simulink model "AAI"  (R2022a)
settings: Solver=FixedStepAuto  StartTime=0.0  StopTime=10.0  FixedStep=1e-3  RelTol=1e-3  EnableMultiTasking=on
undefined symbols (not defined in the file): D0, D10, D11, D12, D13, D2, D4, D5, D6, D7, D8, D9, PTA0, PTA2, PTB23, PTB9, PTC16, PTC2, PTC3, PTC4, PTD0, PTD1, PTD2, PTD3
libraries: frdmk64flib x12
settings Model: ExtModeTrigDuration=5  Creator=ethan  LastModifiedBy=taimu
settings OptimizationCC: EnhancedBackFolding=on  PassReuseOutputArgsAs=Individual arguments  ZeroExternalMemoryAtStartup=off  ZeroInternalMemoryAtStartup=off  MaxStackSize=64  OptimizeBlockOrder=speed  DifferentSizesBufferReuse=on  OptimizationCustomize=off  EfficientTunableParamExpr=on
settings DebuggingCC: ParameterTunabilityLossMsg=error
settings HardwareCC: ProdBitPerPointer=32  ProdBitPerSizeT=32  ProdBitPerPtrDiffT=32  ProdLargestAtomicInteger=Long  ProdLargestAtomicFloat=Double  ProdWordSize=32  ProdHWDeviceType=ARM Compatible->ARM Cortex
settings SFSimCC: MATLABDynamicMemAlloc=off
settings RTWCC: SystemTargetFile=ert.tlc  HardwareBoard=NXP FRDM-K64F  TLCOptions="-aInlineSetEventsForThisBaseRateFcn=TLC_FALSE -aSuppressMultiTaskScheduler=TLC_FALSE  -aRateBasedStepFcn=0"  TemplateMakefile=ert_default_tmf  Toolchain=GNU Tools for ARM Embedded Processors
settings CodeAppCC: ForceParamTrailComments=on  IgnoreCustomStorageClasses=off  OperatorAnnotations=on  SimulinkDataObjDesc=on  SFDataObjDesc=on  InsertBlockDesc=on
settings ERTTargetCC: ExtModeTransport=4  ExtModeMexFile=sendToCommService

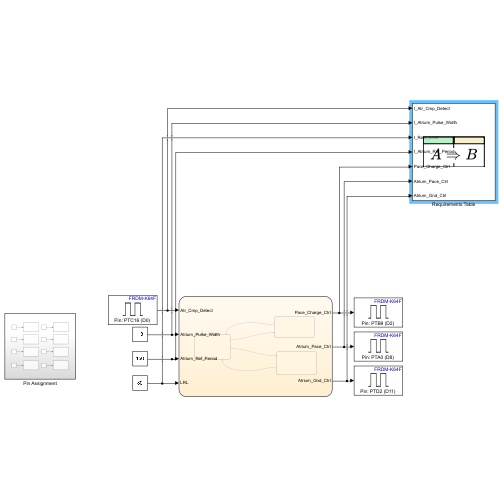
[thumbnail: Simulink's stored preview of the top-level diagram]
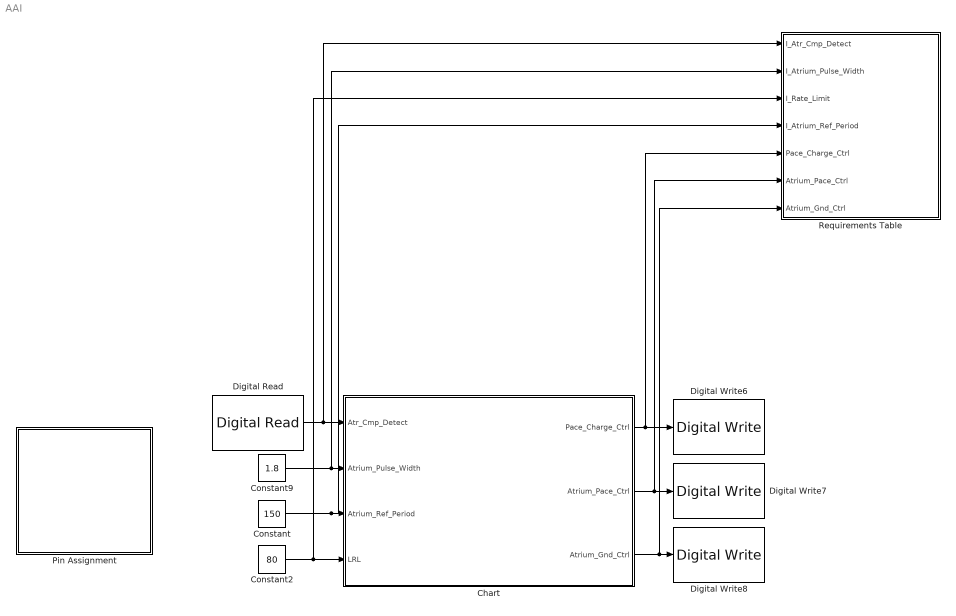
== system AAI ==
  Chart : Stateflow chart  TreatAsAtomicUnit=on
  Constant : Constant  Value=150  OutDataTypeStr=int16
  Constant2 : Constant  Value=80
  Constant9 : Constant  Value=1.8
  Digital Read : frdmk64flib/Digital Read  Whichpin=PTC16 (D0)  SampleTime=-1
  Digital Write6 : frdmk64flib/Digital Write  Whichpin=PTB9 (D2)
  Digital Write7 : frdmk64flib/Digital Write  Whichpin=PTA0 (D8)
  Digital Write8 : frdmk64flib/Digital Write  Whichpin=PTD2 (D11)
  Pin Assignment : Subsystem
  Requirements Table : Requirements Table  TreatAsAtomicUnit=on
  wires:
  Chart/3(Atrium_Gnd_Ctrl) -> Requirements Table/7(Atrium_Gnd_Ctrl), Digital Write8/1
  Chart/2(Atrium_Pace_Ctrl) -> Requirements Table/6(Atrium_Pace_Ctrl), Digital Write7/1
  Constant2/1 -> Requirements Table/3(I_Rate_Limit), Chart/4(LRL)
  Constant9/1 -> Requirements Table/2(I_Atrium_Pulse_Width), Chart/2(Atrium_Pulse_Width)
  Chart/1(Pace_Charge_Ctrl) -> Requirements Table/5(Pace_Charge_Ctrl), Digital Write6/1
  Digital Read/1 -> Requirements Table/1(I_Atr_Cmp_Detect), Chart/1(Atr_Cmp_Detect)
  Constant/1 -> Requirements Table/4(I_Atrium_Ref_Period), Chart/3(Atrium_Ref_Period)

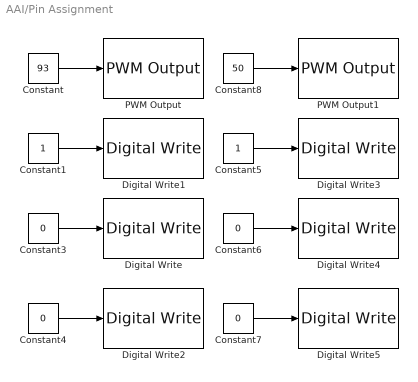
== system AAI/Pin Assignment ==
  Constant : Constant  Value=93  OutDataTypeStr=int8
  Constant1 : Constant
  Constant{3..4,6..7} (4 alike) : Constant  Value=0
  Constant5 : Constant
  Constant8 : Constant  Value=50  OutDataTypeStr=int8
  Digital Write : frdmk64flib/Digital Write  Whichpin=PTB23 (D4)
  Digital Write1 : frdmk64flib/Digital Write  Whichpin=PTD1 (D13)
  Digital Write2 : frdmk64flib/Digital Write  Whichpin=PTC3 (D7)
  Digital Write3 : frdmk64flib/Digital Write  Whichpin=PTD0 (D10)
  Digital Write4 : frdmk64flib/Digital Write  Whichpin=PTD3 (D12)
  Digital Write5 : frdmk64flib/Digital Write  Whichpin=PTC4 (D9)
  PWM Output : frdmk64flib/PWM Output  Whichpin=PTC2 (D6)  InitialFrequency=2000  InitialDutyCycle=0
  PWM Output1 : frdmk64flib/PWM Output  Whichpin=PTA2 (D5)  InitialFrequency=2000  InitialDutyCycle=0
  wires:
  Constant1/1 -> Digital Write1/1
  Constant5/1 -> Digital Write3/1
  Constant7/1 -> Digital Write5/1
  Constant4/1 -> Digital Write2/1
  Constant/1 -> PWM Output/1
  Constant8/1 -> PWM Output1/1
  Constant3/1 -> Digital Write/1
  Constant6/1 -> Digital Write4/1

== stateflow chart AAI/Requirements Table ==
  (default) -> (junction 1073742126)
  (junction 1073742126) -> (junction 1073742127) : {
      | % SF_REQ_REV_07
      | }
  (junction 1073742127) -> (junction 1073742129) : {
      | % HEADER_ASSIGNMENTS
      |
      | }
  (junction 1073742129) -> (junction 1073742131) : {
      | % START_A_4
      | }
  (junction 1073742131) -> (junction 1073742133) : {
      | }
  (junction 1073742133) -> (junction 1073742135)
  (junction 1073742135) -> (junction 1073742137) : {
      | }
  (junction 1073742137) -> (junction 1073742139) : {
      | % END_A_4
      | }
  (junction 1073742139) -> (junction 1073742212) : {
      | % START_R_10
      | }
  (junction 1073742212) -> (junction 1073742214) : {
      | }
  (junction 1073742214) -> (junction 1073742216)
  (junction 1073742216) -> (junction 1073742218) [order 1] : [(((I_Atrium_Pulse_Width) == (0.05)) || ((I_Atrium_Pulse_Width) == (0.1)) || ((I_Atrium_Pulse_Width) == (0.2)) || ((I_Atrium_Pulse_Width) == (0.3)) || ((I_Atrium_Pulse_Width) == (0.4)) || ((I_Atrium_Pulse_Width) == (0.5)) || ((I_Atrium_Pulse_Width) == (0.6)) || ((I_Atrium_Pulse_Width) == (0.7)) || ((I_Atrium_Pulse_Width) == (0.8)) || ((I_Atrium_Pulse_Width) == (0.9)) || ((I_Atrium_Pulse_Width) == (1)) || ((I_Atrium_Pulse_Width) == (1.1)) || ((I_Atrium_Pulse_Width) == (1.2)) || ((I_Atrium_Pulse_Width) == (1.3)) || ((I_Atrium_Pulse_Width) == (1.4)) || ((I_Atrium_Pulse_Width) == (1.5)) || ((I_Atrium_Pulse_Width) == (1.6)) || ((I_Atrium_Pulse_Width) == (1.7)) || ((I_Atrium_Pulse_Width) == (1.8)) || ((I_Atrium_Pulse_Width) == (1.9)) || ((I_Atrium_Pulse_Width) == (20))) && (((I_Rate_Limit) == (30)) || ((I_Rate_Limit) == (35)) || ((I_Rate_Limit) == (40)) || ((I_Rate_Limit) == (45)) || ((I_Rate_Limit) == (50)) || ((I_Rate_Limit) == (51)) || ((I_Rate_Limit) == (52)) || ((I_Rate_Limit) == (53)) || ((I_Rate_Limit) == (54)) || ((I_Rate_Limit) == (55)) || ((I_Rate_Limit) == (56)) || ((I_Rate_Limit) == (57)) || ((I_Rate_Limit) == (58)) || ((I_Rate_Limit) == (59)) || ((I_Rate_Limit) == (60)) || ((I_Rate_Limit) == (61)) || ((I_Rate_Limit) == (62)) || ((I_Rate_Limit) == (63)) || ((I_Rate_Limit) == (64)) || ((I_Rate_Limit) == (65)) || ((I_Rate_Limit) == (66)) || ((I_Rate_Limit) == (67)) || ((I_Rate_Limit) == (68)) || ((I_Rate_Limit) == (69)) || ((I_Rate_Limit) == (70)) || ((I_Rate_Limit) == (71)) || ((I_Rate_Limit) == (72)) || ((I_Rate_Limit) == (73)) || ((I_Rate_Limit) == (74)) || ((I_Rate_Limit) == (75)) || ((I_Rate_Limit) == (76)) || ((I_Rate_Limit) == (77)) || ((I_Rate_Limit) == (78)) || ((I_Rate_Limit) == (79)) || ((I_Rate_Limit) == (80)) || ((I_Rate_Limit) == (81)) || ((I_Rate_Limit) == (82)) || ((I_Rate_Limit) == (83)) || ((I_Rate_Limit) == (84)) || ((I_Rate_Limit) == (85)) || ((I_Rate_Limit) == (86)) || ((I_Rate_Limit) == (87)) || ((I_Rate_Limit) == (88)) || ((I_Rate_Limit) == (89)) || ((I_Rate_Limit) == (90)) || ((I_Rate_Limit) == (95)) || ((I_Rate_Limit) == (100)) || ((I_Rate_Limit) == (105)) || ((I_Rate_Limit) == (110)) || ((I_Rate_Limit) == (115)) || ((I_Rate_Limit) == (120)) || ((I_Rate_Limit) == (125)) || ((I_Rate_Limit) == (130)) || ((I_Rate_Limit) == (135)) || ((I_Rate_Limit) == (140)) || ((I_Rate_Limit) == (145)) || ((I_Rate_Limit) == (150)) || ((I_Rate_Limit) == (155)) || ((I_Rate_Limit) == (160)) || ((I_Rate_Limit) == (165)) || ((I_Rate_Limit) == (170)) || ((I_Rate_Limit) == (175))) && (((I_Atrium_Ref_Period) == (150)) || ((I_Atrium_Ref_Period) == (160)) || ((I_Atrium_Ref_Period) == (170)) || ((I_Atrium_Ref_Period) == (180)) || ((I_Atrium_Ref_Period) == (190)) || ((I_Atrium_Ref_Period) == (200)) || ((I_Atrium_Ref_Period) == (210)) || ((I_Atrium_Ref_Period) == (220)) || ((I_Atrium_Ref_Period) == (230)) || ((I_Atrium_Ref_Period) == (240)) || ((I_Atrium_Ref_Period) == (250)) || ((I_Atrium_Ref_Period) == (260)) || ((I_Atrium_Ref_Period) == (270)) || ((I_Atrium_Ref_Period) == (280)) || ((I_Atrium_Ref_Period) == (290)) || ((I_Atrium_Ref_Period) == (300)) || ((I_Atrium_Ref_Period) == (310)) || ((I_Atrium_Ref_Period) == (320)) || ((I_Atrium_Ref_Period) == (330)) || ((I_Atrium_Ref_Period) == (340)) || ((I_Atrium_Ref_Period) == (350)) || ((I_Atrium_Ref_Period) == (360)) || ((I_Atrium_Ref_Period) == (370)) || ((I_Atrium_Ref_Period) == (380)) || ((I_Atrium_Ref_Period) == (390)) || ((I_Atrium_Ref_Period) == (400)) || ((I_Atrium_Ref_Period) == (410)) || ((I_Atrium_Ref_Period) == (420)) || ((I_Atrium_Ref_Period) == (430)) || ((I_Atrium_Ref_Period) == (440)) || ((I_Atrium_Ref_Period) == (450)) || ((I_Atrium_Ref_Period) == (460)) || ((I_Atrium_Ref_Period) == (470)) || ((I_Atrium_Ref_Period) == (480)) || ((I_Atrium_Ref_Period) == (490)) || ((I_Atrium_Ref_Period) == (500))) && (((I_Atr_Cmp_Detect) == (true)))]
  (junction 1073742216) -> (junction 1073742224) [order 2]
  (junction 1073742218) -> (junction 1073742220) : {
      | reqtable_postcondition(((Pace_Charge_Ctrl == true && Atrium_Gnd_Ctrl == true && Atrium_Pace_Ctrl == false)), 'R:1');
      |
      |
      | }
  (junction 1073742220) -> (junction 1073742222) : {
      | }
  (junction 1073742222) -> (junction 1073742224)
  (junction 1073742224) -> (junction 1073742226)
  (junction 1073742226) -> (junction 1073742228) : {
      | % END_R_10
      | }
  (junction 1073742228) -> (junction 1073742191) : {
      | % START_R_1
      | }
  (junction 1073742191) -> (junction 1073742193) : {
      | }
  (junction 1073742193) -> (junction 1073742195)
  (junction 1073742195) -> (junction 1073742197) [order 1] : [(((I_Atrium_Pulse_Width) == (0.05)) || ((I_Atrium_Pulse_Width) == (0.1)) || ((I_Atrium_Pulse_Width) == (0.2)) || ((I_Atrium_Pulse_Width) == (0.3)) || ((I_Atrium_Pulse_Width) == (0.4)) || ((I_Atrium_Pulse_Width) == (0.5)) || ((I_Atrium_Pulse_Width) == (0.6)) || ((I_Atrium_Pulse_Width) == (0.7)) || ((I_Atrium_Pulse_Width) == (0.8)) || ((I_Atrium_Pulse_Width) == (0.9)) || ((I_Atrium_Pulse_Width) == (1)) || ((I_Atrium_Pulse_Width) == (1.1)) || ((I_Atrium_Pulse_Width) == (1.2)) || ((I_Atrium_Pulse_Width) == (1.3)) || ((I_Atrium_Pulse_Width) == (1.4)) || ((I_Atrium_Pulse_Width) == (1.5)) || ((I_Atrium_Pulse_Width) == (1.6)) || ((I_Atrium_Pulse_Width) == (1.7)) || ((I_Atrium_Pulse_Width) == (1.8)) || ((I_Atrium_Pulse_Width) == (1.9))) && (((I_Rate_Limit) == (30)) || ((I_Rate_Limit) == (35)) || ((I_Rate_Limit) == (40)) || ((I_Rate_Limit) == (45)) || ((I_Rate_Limit) == (50)) || ((I_Rate_Limit) == (51)) || ((I_Rate_Limit) == (52)) || ((I_Rate_Limit) == (53)) || ((I_Rate_Limit) == (54)) || ((I_Rate_Limit) == (55)) || ((I_Rate_Limit) == (56)) || ((I_Rate_Limit) == (57)) || ((I_Rate_Limit) == (58)) || ((I_Rate_Limit) == (59)) || ((I_Rate_Limit) == (60)) || ((I_Rate_Limit) == (61)) || ((I_Rate_Limit) == (62)) || ((I_Rate_Limit) == (63)) || ((I_Rate_Limit) == (64)) || ((I_Rate_Limit) == (65)) || ((I_Rate_Limit) == (66)) || ((I_Rate_Limit) == (67)) || ((I_Rate_Limit) == (68)) || ((I_Rate_Limit) == (69)) || ((I_Rate_Limit) == (70)) || ((I_Rate_Limit) == (71)) || ((I_Rate_Limit) == (72)) || ((I_Rate_Limit) == (73)) || ((I_Rate_Limit) == (74)) || ((I_Rate_Limit) == (75)) || ((I_Rate_Limit) == (76)) || ((I_Rate_Limit) == (77)) || ((I_Rate_Limit) == (78)) || ((I_Rate_Limit) == (79)) || ((I_Rate_Limit) == (80)) || ((I_Rate_Limit) == (81)) || ((I_Rate_Limit) == (82)) || ((I_Rate_Limit) == (83)) || ((I_Rate_Limit) == (84)) || ((I_Rate_Limit) == (85)) || ((I_Rate_Limit) == (86)) || ((I_Rate_Limit) == (87)) || ((I_Rate_Limit) == (88)) || ((I_Rate_Limit) == (89)) || ((I_Rate_Limit) == (90)) || ((I_Rate_Limit) == (95)) || ((I_Rate_Limit) == (100)) || ((I_Rate_Limit) == (105)) || ((I_Rate_Limit) == (110)) || ((I_Rate_Limit) == (115)) || ((I_Rate_Limit) == (120)) || ((I_Rate_Limit) == (125)) || ((I_Rate_Limit) == (130)) || ((I_Rate_Limit) == (135)) || ((I_Rate_Limit) == (140)) || ((I_Rate_Limit) == (145)) || ((I_Rate_Limit) == (150)) || ((I_Rate_Limit) == (155)) || ((I_Rate_Limit) == (160)) || ((I_Rate_Limit) == (165)) || ((I_Rate_Limit) == (170)) || ((I_Rate_Limit) == (175))) && (((I_Atrium_Ref_Period) == (150)) || ((I_Atrium_Ref_Period) == (160)) || ((I_Atrium_Ref_Period) == (170)) || ((I_Atrium_Ref_Period) == (180)) || ((I_Atrium_Ref_Period) == (190)) || ((I_Atrium_Ref_Period) == (200)) || ((I_Atrium_Ref_Period) == (210)) || ((I_Atrium_Ref_Period) == (220)) || ((I_Atrium_Ref_Period) == (230)) || ((I_Atrium_Ref_Period) == (240)) || ((I_Atrium_Ref_Period) == (250)) || ((I_Atrium_Ref_Period) == (260)) || ((I_Atrium_Ref_Period) == (270)) || ((I_Atrium_Ref_Period) == (280)) || ((I_Atrium_Ref_Period) == (290)) || ((I_Atrium_Ref_Period) == (300)) || ((I_Atrium_Ref_Period) == (310)) || ((I_Atrium_Ref_Period) == (320)) || ((I_Atrium_Ref_Period) == (330)) || ((I_Atrium_Ref_Period) == (340)) || ((I_Atrium_Ref_Period) == (350)) || ((I_Atrium_Ref_Period) == (360)) || ((I_Atrium_Ref_Period) == (370)) || ((I_Atrium_Ref_Period) == (380)) || ((I_Atrium_Ref_Period) == (390)) || ((I_Atrium_Ref_Period) == (400)) || ((I_Atrium_Ref_Period) == (410)) || ((I_Atrium_Ref_Period) == (420)) || ((I_Atrium_Ref_Period) == (430)) || ((I_Atrium_Ref_Period) == (440)) || ((I_Atrium_Ref_Period) == (450)) || ((I_Atrium_Ref_Period) == (460)) || ((I_Atrium_Ref_Period) == (470)) || ((I_Atrium_Ref_Period) == (480)) || ((I_Atrium_Ref_Period) == (490)) || ((I_Atrium_Ref_Period) == (500))) && (((I_Atr_Cmp_Detect) == (false)))]
  (junction 1073742195) -> (junction 1073742203) [order 2]
  (junction 1073742197) -> (junction 1073742199) : {
      | reqtable_postcondition(((Pace_Charge_Ctrl == true && Atrium_Gnd_Ctrl == true && Atrium_Pace_Ctrl == false) || (Pace_Charge_Ctrl == false && Atrium_Gnd_Ctrl == false && Atrium_Pace_Ctrl == true)), 'R:2');
      |
      |
      | }
  (junction 1073742199) -> (junction 1073742201) : {
      | }
  (junction 1073742201) -> (junction 1073742203)
  (junction 1073742203) -> (junction 1073742205)
  (junction 1073742205) -> (junction 1073742207) : {
      | % END_R_1
      | }
  data: I_Atr_Cmp_Detect input; I_Atrium_Pulse_Width input; I_Rate_Limit input; I_Atrium_Ref_Period input; Pace_Charge_Ctrl input; Atrium_Pace_Ctrl input; Atrium_Gnd_Ctrl input

== stateflow chart AAI/Chart ==
  state Inhibit
    entry:
    Atrium_Pace_Ctrl = false;
    Atrium_Gnd_Ctrl = true;
    Pace_Charge_Ctrl = true;
  state Signal_Search
    entry:
    Atrium_Pace_Ctrl = false;
    Atrium_Gnd_Ctrl = true;
    Pace_Charge_Ctrl = true;
  state Pace
    entry:
    Pace_Charge_Ctrl = false;
    Atrium_Pace_Ctrl = true;
    Atrium_Gnd_Ctrl = false;
  Inhibit -> Signal_Search : after(Atrium_Ref_Period,msec)
  (default) -> Signal_Search
  Signal_Search -> Inhibit [order 2] : [Atr_Cmp_Detect == true]
  Signal_Search -> Pace [order 1] : [after(((60000/LRL)-Atrium_Pulse_Width),msec)]
  Pace -> Signal_Search : after(Atrium_Pulse_Width,msec)
  data: Atr_Cmp_Detect input boolean; Atrium_Pulse_Width input; Atrium_Ref_Period input; Pace_Charge_Ctrl output; Atrium_Pace_Ctrl output; Atrium_Gnd_Ctrl output; LRL input
